simulink model "PID_MoreJoints1_6"  (R2018b)
settings: Solver=FixedStepDiscrete  StartTime=0.0  StopTime=Inf  FixedStep=0.001  RelTol=1e-3  EnableMultiTasking=on
undefined symbols (not defined in the file): DiscIntNeverNeededParam, J1, J2, J3, J4, J5, J6, J7, Motor_Current, Motor_Position, Motor_Velocity, q, qd, Send_GUIdata, Tau
libraries: c280xlib x14, simulink x11, dspsrcs4 x6, idelinklib_common x1
(part 1 of 4)
settings Model: ExtModeTrigDuration=8  Creator=Administrator  LastModifiedBy=Jeason
settings OptimizationCC: DefaultUnderspecifiedDataType=single  EnhancedBackFolding=on  PassReuseOutputArgsAs=Individual arguments  MaxStackSize=512  OptimizeBlockOrder=speed  DifferentSizesBufferReuse=on  OptimizationCustomize=off
settings DebuggingCC: InheritedTsInSrcMsg=none  MultiTaskDSMMsg=none  ParameterTunabilityLossMsg=error
settings HardwareCC: ProdBitPerChar=16  ProdBitPerInt=16  ProdBitPerPointer=32  ProdBitPerSizeT=32  ProdBitPerPtrDiffT=32  ProdLargestAtomicInteger=Integer  ProdLargestAtomicFloat=None  ProdWordSize=16  ProdLongLongMode=on  ProdHWDeviceType=Texas Instruments->C2000
settings SFSimCC: MATLABDynamicMemAlloc=off
settings RTWCC: SystemTargetFile=ert.tlc  HardwareBoard=TI Delfino F2833x  TemplateMakefile=ert_default_tmf  GenerateReport=on  Toolchain=Texas Instruments Code Composer Studio (C2000)  IncludeHyperlinkInReport=on  LaunchReport=on  GenerateTraceInfo=on  GenerateTraceReport=on  GenerateTraceReportSl=on  GenerateTraceReportSf=on  GenerateTraceReportEml=on
settings CodeAppCC: ForceParamTrailComments=on  IgnoreCustomStorageClasses=off  OperatorAnnotations=on  SimulinkDataObjDesc=on  SFDataObjDesc=on  InsertBlockDesc=on
settings ERTTargetCC: CodeReplacementLibrary=TI C28x

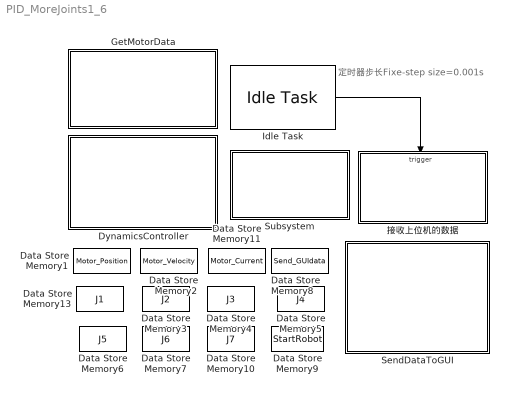
== system PID_MoreJoints1_6 ==
  note: 定时器步长Fixe-step size=0.001s
  Data Store Memory1 : DataStoreMemory  DataStoreName=Motor_Position  ReadBeforeWriteMsg=warning  WriteAfterWriteMsg=warning  WriteAfterReadMsg=warning  InitialValue=[0 0 0 0 0 0]  ShowAdditionalParam=off  OutDataTypeStr=int32
      settings: RTWStateStorageClass=ExportedGlobal
  Data Store Memory10 : DataStoreMemory  DataStoreName=J7  ReadBeforeWriteMsg=warning  WriteAfterWriteMsg=warning  WriteAfterReadMsg=warning  InitialValue=[0 0 0 0 0 0]  ShowAdditionalParam=off  OutDataTypeStr=double
      settings: RTWStateStorageClass=ExportedGlobal
  Data Store Memory11 : DataStoreMemory  DataStoreName=Motor_Current  ReadBeforeWriteMsg=warning  WriteAfterWriteMsg=warning  WriteAfterReadMsg=warning  InitialValue=[0 0 0 0 0 0]  ShowAdditionalParam=off  OutDataTypeStr=int32
      settings: RTWStateStorageClass=ExportedGlobal
  Data Store Memory13 : DataStoreMemory  DataStoreName=J1  ReadBeforeWriteMsg=warning  WriteAfterWriteMsg=warning  WriteAfterReadMsg=warning  InitialValue=[0 0 0 0 0 0]  ShowAdditionalParam=off  OutDataTypeStr=double
      settings: RTWStateStorageClass=ExportedGlobal
  Data Store Memory2 : DataStoreMemory  DataStoreName=Motor_Velocity  ReadBeforeWriteMsg=warning  WriteAfterWriteMsg=warning  WriteAfterReadMsg=warning  InitialValue=[0 0 0 0 0 0]  ShowAdditionalParam=off  OutDataTypeStr=int32
      settings: RTWStateStorageClass=ExportedGlobal
  Data Store Memory3 : DataStoreMemory  DataStoreName=J2  ReadBeforeWriteMsg=warning  WriteAfterWriteMsg=warning  WriteAfterReadMsg=warning  InitialValue=[0 0 0 0 0 0]  ShowAdditionalParam=off  OutDataTypeStr=double
      settings: RTWStateStorageClass=ExportedGlobal
  Data Store Memory4 : DataStoreMemory  DataStoreName=J3  ReadBeforeWriteMsg=warning  WriteAfterWriteMsg=warning  WriteAfterReadMsg=warning  InitialValue=[0 0 0 0 0 0]  ShowAdditionalParam=off  OutDataTypeStr=double
      settings: RTWStateStorageClass=ExportedGlobal
  Data Store Memory5 : DataStoreMemory  DataStoreName=J4  ReadBeforeWriteMsg=warning  WriteAfterWriteMsg=warning  WriteAfterReadMsg=warning  InitialValue=[0 0 0 0 0 0]  ShowAdditionalParam=off  OutDataTypeStr=double
      settings: RTWStateStorageClass=ExportedGlobal
  Data Store Memory6 : DataStoreMemory  DataStoreName=J5  ReadBeforeWriteMsg=warning  WriteAfterWriteMsg=warning  WriteAfterReadMsg=warning  InitialValue=[0 0 0 0 0 0]  ShowAdditionalParam=off  OutDataTypeStr=double
      settings: RTWStateStorageClass=ExportedGlobal
  Data Store Memory7 : DataStoreMemory  DataStoreName=J6  ReadBeforeWriteMsg=warning  WriteAfterWriteMsg=warning  WriteAfterReadMsg=warning  InitialValue=[0 0 0 0 0 0]  ShowAdditionalParam=off  OutDataTypeStr=double
      settings: RTWStateStorageClass=ExportedGlobal
  Data Store Memory8 : DataStoreMemory  DataStoreName=Send_GUIdata  ReadBeforeWriteMsg=warning  WriteAfterWriteMsg=warning  WriteAfterReadMsg=warning  InitialValue=zeros(1,18)  ShowAdditionalParam=off  OutDataTypeStr=double
      settings: RTWStateStorageClass=ExportedGlobal
  Data Store Memory9 : DataStoreMemory  DataStoreName=StartRobot  ReadBeforeWriteMsg=warning  WriteAfterWriteMsg=warning  WriteAfterReadMsg=warning  ShowAdditionalParam=off  OutDataTypeStr=uint16
      settings: RTWStateStorageClass=ExportedGlobal
  DynamicsController : Subsystem  Tag=Calculated_Data  Priority=2  TreatAsAtomicUnit=on  RTWFcnName=DynamicsController
      settings: RTWSystemCode=Nonreusable function  RTWFcnNameOpts=User specified  RTWFileNameOpts=Use function name
      mask Display:
      | color('red')
      | disp('六轴多关节\nPID算法动力学控制')
  GetMotorData : Subsystem  Tag=Get_Data  Priority=0  TreatAsAtomicUnit=on
      settings: RTWSystemCode=Nonreusable function
  Idle Task : idelinklib_common/Idle Task  tasknumbers=[0]  taskpriorities=100016  taskpreempts=[1]  showinput=off  simPriority=0
  SendDataToGUI : Subsystem  Priority=2  TreatAsAtomicUnit=on
      settings: RTWSystemCode=Nonreusable function
  Subsystem : Subsystem
      mask Display: disp('System\nInitialization');
  接收上位机的数据 : Subsystem  TreatAsAtomicUnit=on
  wires:
  Idle Task/1 -> 接收上位机的数据/Trigger

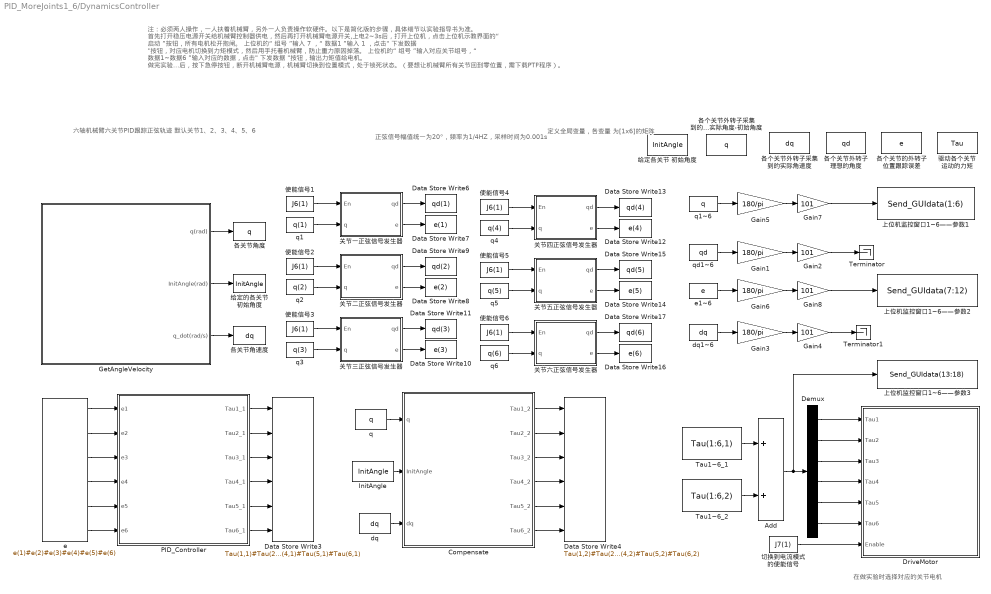
== system PID_MoreJoints1_6/DynamicsController ==
  note: 定义全局变量，各变量
      | 为[1x6]的矩阵
  note: 六轴机械臂六关节PID跟踪正弦轨迹
      | 默认关节1、2、3、4、5、6
  note: 在做实验时选择对应的关节电机
  note: 正弦信号幅值统一为20°，频率为1/4HZ，采样时间为0.001s
  note: 注：必须两人操作，一人扶着机械臂，另外一人负责操作软硬件。以下是简化版的步骤，具体细节以实验指导书为准。
      | 首先打开稳压电源开关给机械臂控制器供电，然后再打开机械臂电源开关,上电2~3s后，打开上位机，点击上位机示教界面的“ 启动 ”按钮，所有电机松开抱闸。
      | 上位机的“ 组号 ”输入 7 ，“ 数据1 ”输入 1 ，点击" 下发数据 "按钮，对应电机切换到力矩模式，然后用手托着机械臂，防止重力原因掉落。
      | 上位机的“ 组号 ”输入对应关节组号，“ 数据1~数据6 ”输入对应的数据，点击" 下发数据 "按钮，输出力矩值给电机。
      | 做完实验后，按下急停按钮，断开机械臂电源，机械臂切换到位置模式，处于锁死状态。（要想让机械臂所有关节回到零位置，需下载PTP程序）。
  Add : Sum
  Compensate : Subsystem  Priority=8  TreatAsAtomicUnit=on  RTWFcnName=Compensate
      settings: RTWSystemCode=Nonreusable function  RTWFcnNameOpts=User specified  RTWFileNameOpts=Use function name
  Data Store Write10 : DataStoreWrite  DataStoreName=e  DataStoreElements=e(3)
  Data Store Write11 : DataStoreWrite  DataStoreName=qd  DataStoreElements=qd(3)
  Data Store Write12 : DataStoreWrite  DataStoreName=e  DataStoreElements=e(4)
  Data Store Write13 : DataStoreWrite  DataStoreName=qd  DataStoreElements=qd(4)
  Data Store Write14 : DataStoreWrite  DataStoreName=e  DataStoreElements=e(5)
  Data Store Write15 : DataStoreWrite  DataStoreName=qd  DataStoreElements=qd(5)
  Data Store Write16 : DataStoreWrite  DataStoreName=e  DataStoreElements=e(6)
  Data Store Write17 : DataStoreWrite  DataStoreName=qd  DataStoreElements=qd(6)
  Data Store Write3 : DataStoreWrite  DataStoreName=Tau  DataStoreElements=Tau(1,1)#Tau(2,1)#Tau(3,1)#Tau(4,1)#Tau(5,1)#Tau(6,1)
  Data Store Write4 : DataStoreWrite  DataStoreName=Tau  DataStoreElements=Tau(1,2)#Tau(2,2)#Tau(3,2)#Tau(4,2)#Tau(5,2)#Tau(6,2)
  Data Store Write6 : DataStoreWrite  DataStoreName=qd  DataStoreElements=qd(1)
  Data Store Write7 : DataStoreWrite  DataStoreName=e  DataStoreElements=e(1)
  Data Store Write8 : DataStoreWrite  DataStoreName=e  DataStoreElements=e(2)
  Data Store Write9 : DataStoreWrite  DataStoreName=qd  DataStoreElements=qd(2)
  Demux : Demux  Outputs=6
  DriveMotor : Subsystem  TreatAsAtomicUnit=on  RTWFcnName=DrivrMotor  mask(DriverMotor){Motor1=on, Motor2=on, Motor3=on, Motor4=on, Motor5=on, Motor6=on}
      mask help:
      | 当其中一个Motor勾选时，表示将力矩输出给对应的电机；如果不勾选时，表示对应的电机不工作。
      | 比如：如果做单关节实验时，哪个电机要做实验就勾选对应的电机，其他电机一定要不勾选。
      | 关节1~3为CANB,关节4~6为CANA,驱动邮箱号为7~12。输入量的范围限定在-900~900。
      settings: RTWSystemCode=Nonreusable function  RTWFcnNameOpts=User specified  RTWFileNameOpts=Use function name
      mask Callback Motor1:
      | vssBlk1 = [gcb, '/BottomDriver/Joint1'];
      | choice1 = get_param(gcb,'Motor1');
      | if strcmp(choice1,'off')
      |         set_param(vssBlk1, 'Commented','on');
      |     else
      |         set_param(vssBlk1, 'Commented','off');
      | end
      | clear choice1 vssBlk1;
      mask Callback Motor2:
      | vssBlk2 = [gcb, '/BottomDriver/Joint2'];
      | choice2 = get_param(gcb,'Motor2');
      | if strcmp(choice2,'off')
      |         set_param(vssBlk2, 'Commented','on');
      |     else
      |         set_param(vssBlk2, 'Commented','off');
      | end
      | clear choice2 vssBlk2;
      mask Callback Motor3:
      | vssBlk3 = [gcb, '/BottomDriver/Joint3'];
      | choice3 = get_param(gcb,'Motor3');
      | if strcmp(choice3,'off')
      |         set_param(vssBlk3, 'Commented','on');
      |     else
      |         set_param(vssBlk3, 'Commented','off');
      | end
      | clear choice3 vssBlk3;
      mask Callback Motor4:
      | vssBlk4 = [gcb, '/BottomDriver/Joint4'];
      | choice4 = get_param(gcb,'Motor4');
      | if strcmp(choice4,'off')
      |         set_param(vssBlk4, 'Commented','on');
      |     else
      |         set_param(vssBlk4, 'Commented','off');
      | end
      | clear choice4 vssBlk4;
      mask Callback Motor5:
      | vssBlk5 = [gcb, '/BottomDriver/Joint5'];
      | choice5 = get_param(gcb,'Motor5');
      | if strcmp(choice5,'off')
      |         set_param(vssBlk5, 'Commented','on');
      |     else
      |         set_param(vssBlk5, 'Commented','off');
      | end
      | clear choice5 vssBlk5;
      mask Callback Motor6:
      | vssBlk6 = [gcb, '/BottomDriver/Joint6'];
      | choice6 = get_param(gcb,'Motor6');
      | if strcmp(choice6,'off')
      |         set_param(vssBlk6, 'Commented','on');
      |     else
      |         set_param(vssBlk6, 'Commented','off');
      | end
      | clear choice6 vssBlk6;
      mask Display:
      | disp('DriverMotor');
      | port_label('input', 1, 'Tau1');
      | port_label('input', 2, 'Tau2');
      | port_label('input', 3, 'Tau3');
      | port_label('input', 4, 'Tau4');
      | port_label('input', 5, 'Tau5');
      | port_label('input', 6, 'Tau6');
      | port_label('input', 7, 'Enable');
  Gain{1,3,5..6} (4 alike) : Gain  Gain=180/pi
  Gain{2,4,7..8} (4 alike) : Gain  Gain=101
  GetAngleVelocity : Subsystem  Priority=0  TreatAsAtomicUnit=on  RTWFcnName=GetAngleVelocity
      settings: RTWSystemCode=Nonreusable function  RTWFcnNameOpts=User specified  RTWFileNameOpts=Use function name
  InitAngle : DataStoreRead  DataStoreName=InitAngle
  PID_Controller : Subsystem  Priority=7  TreatAsAtomicUnit=on  RTWFcnName=PID_Controller
      settings: RTWSystemCode=Nonreusable function  RTWFcnNameOpts=User specified  RTWFileNameOpts=Use function name
  Tau1~6_1 : DataStoreRead  DataStoreName=Tau  DataStoreElements=Tau(1:6,1)
  Tau1~6_2 : DataStoreRead  DataStoreName=Tau  DataStoreElements=Tau(1:6,2)
  Terminator : Terminator
  Terminator1 : Terminator
  dq : DataStoreRead  DataStoreName=dq
  dq1~6 : DataStoreRead  DataStoreName=dq
  e : DataStoreRead  DataStoreName=e  DataStoreElements=e(1)#e(2)#e(3)#e(4)#e(5)#e(6)
  e1~6 : DataStoreRead  DataStoreName=e
  q : DataStoreRead  DataStoreName=q
  q1 : DataStoreRead  DataStoreName=q  DataStoreElements=q(1)
  q1~6 : DataStoreRead  DataStoreName=q
  q2 : DataStoreRead  DataStoreName=q  DataStoreElements=q(2)
  q3 : DataStoreRead  DataStoreName=q  DataStoreElements=q(3)
  q4 : DataStoreRead  DataStoreName=q  DataStoreElements=q(4)
  q5 : DataStoreRead  DataStoreName=q  DataStoreElements=q(5)
  q6 : DataStoreRead  DataStoreName=q  DataStoreElements=q(6)
  qd1~6 : DataStoreRead  DataStoreName=qd
  上位机监控窗口1~6——参数1 : DataStoreWrite  DataStoreName=Send_GUIdata  DataStoreElements=Send_GUIdata(1:6)
  上位机监控窗口1~6——参数2 : DataStoreWrite  DataStoreName=Send_GUIdata  DataStoreElements=Send_GUIdata(7:12)
  上位机监控窗口1~6——参数3 : DataStoreWrite  DataStoreName=Send_GUIdata  DataStoreElements=Send_GUIdata(13:18)
  使能信号{1..6} (6 alike) : DataStoreRead  DataStoreName=J6  DataStoreElements=J6(1)
  关节一正弦信号发生器 : Subsystem  Priority=1  TreatAsAtomicUnit=on  RTWFcnName=SineSignal
      settings: RTWFcnNameOpts=User specified  RTWFileNameOpts=Use function name
  关节三正弦信号发生器 : Subsystem  Priority=3  TreatAsAtomicUnit=on  RTWFcnName=SineSignal
      settings: RTWFcnNameOpts=User specified  RTWFileNameOpts=Use function name
  关节二正弦信号发生器 : Subsystem  Priority=2  TreatAsAtomicUnit=on  RTWFcnName=SineSignal
      settings: RTWFcnNameOpts=User specified  RTWFileNameOpts=Use function name
  关节五正弦信号发生器 : Subsystem  Priority=5  TreatAsAtomicUnit=on  RTWFcnName=SineSignal
      settings: RTWFcnNameOpts=User specified  RTWFileNameOpts=Use function name
  关节六正弦信号发生器 : Subsystem  Priority=6  TreatAsAtomicUnit=on  RTWFcnName=SineSignal
      settings: RTWFcnNameOpts=User specified  RTWFileNameOpts=Use function name
  关节四正弦信号发生器 : Subsystem  Priority=4  TreatAsAtomicUnit=on  RTWFcnName=SineSignal
      settings: RTWFcnNameOpts=User specified  RTWFileNameOpts=Use function name
  切换到电流模式 的使能信号 : DataStoreRead  DataStoreName=J7  DataStoreElements=J7(1)
  各个关节外转子 理想的角度 : DataStoreMemory  DataStoreName=qd  ReadBeforeWriteMsg=warning  WriteAfterWriteMsg=warning  WriteAfterReadMsg=warning  InitialValue=zeros(1,6)  ShowAdditionalParam=off  OutDataTypeStr=double
      settings: RTWStateStorageClass=ExportedGlobal
  各个关节外转子采集 到的实际角度-初始角度 : DataStoreMemory  DataStoreName=q  ReadBeforeWriteMsg=warning  WriteAfterWriteMsg=warning  WriteAfterReadMsg=warning  InitialValue=zeros(1,6)  ShowAdditionalParam=off  OutDataTypeStr=double
      settings: RTWStateStorageClass=ExportedGlobal
  各个关节外转子采集 到的实际角速度 : DataStoreMemory  DataStoreName=dq  ReadBeforeWriteMsg=warning  WriteAfterWriteMsg=warning  WriteAfterReadMsg=warning  InitialValue=zeros(1,6)  ShowAdditionalParam=off  OutDataTypeStr=double
      settings: RTWStateStorageClass=ExportedGlobal
  各个关节的外转子 位置跟踪误差 : DataStoreMemory  DataStoreName=e  ReadBeforeWriteMsg=warning  WriteAfterWriteMsg=warning  WriteAfterReadMsg=warning  InitialValue=zeros(1,6)  ShowAdditionalParam=off  OutDataTypeStr=double
      settings: RTWStateStorageClass=ExportedGlobal
  各关节角度 : DataStoreWrite  DataStoreName=q
  各关节角速度 : DataStoreWrite  DataStoreName=dq
  给定各关节 初始角度 : DataStoreMemory  DataStoreName=InitAngle  ReadBeforeWriteMsg=warning  WriteAfterWriteMsg=warning  WriteAfterReadMsg=warning  InitialValue=zeros(1,6)  ShowAdditionalParam=off  OutDataTypeStr=double
      settings: RTWStateStorageClass=ExportedGlobal
  给定的各关节 初始角度 : DataStoreWrite  DataStoreName=InitAngle
  驱动各个关节 运动的力矩 : DataStoreMemory  DataStoreName=Tau  ReadBeforeWriteMsg=warning  WriteAfterWriteMsg=warning  WriteAfterReadMsg=warning  InitialValue=zeros(6,2)  ShowAdditionalParam=off  OutDataTypeStr=double
      settings: RTWStateStorageClass=ExportedGlobal
  wires:
  使能信号1/1 -> 关节一正弦信号发生器/1(En)
  使能信号2/1 -> 关节二正弦信号发生器/1(En)
  使能信号3/1 -> 关节三正弦信号发生器/1(En)
  使能信号4/1 -> 关节四正弦信号发生器/1(En)
  使能信号5/1 -> 关节五正弦信号发生器/1(En)
  使能信号6/1 -> 关节六正弦信号发生器/1(En)
  关节一正弦信号发生器/1(qd) -> Data Store Write6/1
  关节二正弦信号发生器/1(qd) -> Data Store Write9/1
  关节三正弦信号发生器/1(qd) -> Data Store Write11/1
  关节四正弦信号发生器/1(qd) -> Data Store Write13/1
  关节五正弦信号发生器/1(qd) -> Data Store Write15/1
  关节六正弦信号发生器/1(qd) -> Data Store Write17/1
  关节一正弦信号发生器/2(e) -> Data Store Write7/1
  关节二正弦信号发生器/2(e) -> Data Store Write8/1
  关节三正弦信号发生器/2(e) -> Data Store Write10/1
  关节四正弦信号发生器/2(e) -> Data Store Write12/1
  关节五正弦信号发生器/2(e) -> Data Store Write14/1
  关节六正弦信号发生器/2(e) -> Data Store Write16/1
  q1/1 -> 关节一正弦信号发生器/2(q)
  q2/1 -> 关节二正弦信号发生器/2(q)
  q3/1 -> 关节三正弦信号发生器/2(q)
  q4/1 -> 关节四正弦信号发生器/2(q)
  q5/1 -> 关节五正弦信号发生器/2(q)
  q6/1 -> 关节六正弦信号发生器/2(q)
  e/1 -> PID_Controller/1(e1)
  e/2 -> PID_Controller/2(e2)
  e/3 -> PID_Controller/3(e3)
  e/4 -> PID_Controller/4(e4)
  e/5 -> PID_Controller/5(e5)
  e/6 -> PID_Controller/6(e6)
  PID_Controller/1(Tau1_1) -> Data Store Write3/1
  PID_Controller/2(Tau2_1) -> Data Store Write3/2
  PID_Controller/3(Tau3_1) -> Data Store Write3/3
  PID_Controller/4(Tau4_1) -> Data Store Write3/4
  PID_Controller/5(Tau5_1) -> Data Store Write3/5
  PID_Controller/6(Tau6_1) -> Data Store Write3/6
  Tau1~6_1/1 -> Add/1
  Tau1~6_2/1 -> Add/2
  Add/1 -> 上位机监控窗口1~6——参数3/1, Demux/1
  Demux/6 -> DriveMotor/6(Tau6)
  Demux/5 -> DriveMotor/5(Tau5)
  Demux/4 -> DriveMotor/4(Tau4)
  Demux/3 -> DriveMotor/3(Tau3)
  Demux/2 -> DriveMotor/2(Tau2)
  Demux/1 -> DriveMotor/1(Tau1)
  切换到电流模式 的使能信号/1 -> DriveMotor/7(Enable)
  q1~6/1 -> Gain5/1
  Gain5/1 -> Gain7/1
  Gain1/1 -> Gain2/1
  qd1~6/1 -> Gain1/1
  Gain3/1 -> Gain4/1
  dq1~6/1 -> Gain3/1
  Gain6/1 -> Gain8/1
  e1~6/1 -> Gain6/1
  Gain7/1 -> 上位机监控窗口1~6——参数1/1
  Gain8/1 -> 上位机监控窗口1~6——参数2/1
  Gain4/1 -> Terminator1/1
  q/1 -> Compensate/1(q)
  dq/1 -> Compensate/3(dq)
  Gain2/1 -> Terminator/1
  Compensate/1(Tau1_2) -> Data Store Write4/1
  Compensate/2(Tau2_2) -> Data Store Write4/2
  Compensate/3(Tau3_2) -> Data Store Write4/3
  Compensate/4(Tau4_2) -> Data Store Write4/4
  Compensate/5(Tau5_2) -> Data Store Write4/5
  Compensate/6(Tau6_2) -> Data Store Write4/6
  GetAngleVelocity/2(InitAngle(rad)) -> 给定的各关节 初始角度/1
  GetAngleVelocity/3(q_dot(rad/s)) -> 各关节角速度/1
  GetAngleVelocity/1(q(rad)) -> 各关节角度/1
  InitAngle/1 -> Compensate/2(InitAngle)

== system PID_MoreJoints1_6/GetMotorData ==
  note: 获取关节电流、 角速度、 角度信息
  CANA_284_24 : Subsystem  Priority=4  TreatAsAtomicUnit=on
      settings: RTWSystemCode=Nonreusable function
      mask Display:
      | color('WHITE')
      | disp('JOINT4\n数据读取')
  CANA_285_25 : Subsystem  Priority=5  TreatAsAtomicUnit=on
      settings: RTWSystemCode=Nonreusable function
      mask Display:
      | color('WHITE')
      | disp('JOINT5\n数据读取')
  CANA_286_26 : Subsystem  Priority=6  TreatAsAtomicUnit=on
      settings: RTWSystemCode=Nonreusable function
      mask Display:
      | color('WHITE')
      | disp('JOINT6\n数据读取')
  CANB_281_21 : Subsystem  Priority=1  TreatAsAtomicUnit=on
      settings: RTWSystemCode=Nonreusable function
      mask Display:
      | color('WHITE')
      | disp('JOINT1\n数据读取')
  CANB_282_22 : Subsystem  Priority=2  TreatAsAtomicUnit=on
      settings: RTWSystemCode=Nonreusable function
      mask Display:
      | color('white')
      | disp('JOINT2\n数据读取')
  CANB_283_23 : Subsystem  Priority=3  TreatAsAtomicUnit=on
      settings: RTWSystemCode=Nonreusable function
      mask Display:
      | color('white')
      | disp('JOINT3\n数据读取')

== system PID_MoreJoints1_6/SendDataToGUI ==
  note: Upper limit=9
  note: 发送数据给上位机
  note: 定时器步长Fixe-step size=0.001s,
      | 每10ms发送一次数据给上位机
  " " : Subsystem
  Constant : Constant  Value=true  OutDataTypeStr=boolean
  Constant1 : Constant  Value=false  OutDataTypeStr=boolean
  Switch : Switch  Criteria=u2 > Threshold
  广播周期 : simulink/Sources/Counter Limited  uplimit=9  tsamp=-1
  wires:
  Switch/1 -> " "/Enable
  广播周期/1 -> Switch/2
  Constant1/1 -> Switch/1
  Constant/1 -> Switch/3

== system PID_MoreJoints1_6/Subsystem ==
  Model Header : Subsystem  mask(Model Header){ShowInLibBrowser=0}
      mask prompts: ShowInLibBrowser "Simulink:masks:CustCodeMaskParam1_MP"
      settings: CopyFcn=cccopyfcn(gcb)  OpenFcn=ccopenfcn('Model Header')
      mask Help: eval('feval(''rtwprivate'',''rtwhelpview'',''rtw_model_header_block'')');
      mask Display: disp('Model\nHeader');
  Model Source : Subsystem  mask(Model Source){ShowInLibBrowser=0}
      mask prompts: ShowInLibBrowser "Simulink:masks:CustCodeMaskParam1_MP"
      settings: CopyFcn=cccopyfcn(gcb)  OpenFcn=ccopenfcn('Model Source')
      mask Help: eval('feval(''rtwprivate'',''rtwhelpview'',''rtw_model_source_block'')');
      mask Display: disp('Model\nSource');
  System Initialize : Subsystem  mask(System Initialize){ShowInLibBrowser=0}
      mask prompts: ShowInLibBrowser "Simulink:masks:CustCodeMaskParam1_MP"
      settings: CopyFcn=cccopyfcn(gcb)  OpenFcn=ccopenfcn('System Initialize Function')
      mask Help: eval('feval(''rtwprivate'',''rtwhelpview'',''rtw_sys_initialize_block'')');
      mask Display: disp('System\nInitialize');

== system PID_MoreJoints1_6/接收上位机的数据 ==
  note: 接收上位机数据
  function : TriggerPort  TriggerType=function-call  VariantControl=Variant
  0x0080 : simulink/Logic and Bit Operations/Compare To Constant  relop===  const=hex2dec('0080')  OutDataTypeStr=boolean
  0x88 : simulink/Logic and Bit Operations/Compare To Constant  relop===  const=hex2dec('0088')  OutDataTypeStr=boolean
  Compare To Constant1 : simulink/Logic and Bit Operations/Compare To Constant  relop===  const=hex2dec('0001')  OutDataTypeStr=boolean
  Compare To Constant2 : simulink/Logic and Bit Operations/Compare To Constant  relop===  const=hex2dec('0001')  OutDataTypeStr=boolean
  Data Store Read : DataStoreRead  DataStoreName=PTX
  Data Store Write2 : DataStoreWrite  DataStoreName=StartRobot
  Data Type Conversion : DataTypeConversion  OutDataTypeStr=int16
  Data Type Conversion3 : DataTypeConversion  OutDataTypeStr=double
  Data Type Conversion4 : DataTypeConversion  OutDataTypeStr=uint16
  Demux1 : Demux  Outputs=9
  Logical Operator : Logic  Inputs=4  AllPortsSameDT=off  OutDataTypeStr=boolean
  Mux1 : Mux  Inputs=6
  Subsystem : Subsystem
  Terminator3 : Terminator
  消息使能 : DataStoreMemory  DataStoreName=PTX  ReadBeforeWriteMsg=warning  WriteAfterWriteMsg=warning  WriteAfterReadMsg=warning  InitialValue=true  ShowAdditionalParam=off  OutDataTypeStr=boolean
  获取用户命令 : Subsystem  Priority=1  TreatAsAtomicUnit=on
      settings: RTWSystemCode=Nonreusable function
  wires:
  Compare To Constant2/1 -> Logical Operator/4
  Compare To Constant1/1 -> Logical Operator/3
  Data Store Read/1 -> Logical Operator/2
  Logical Operator/1 -> Data Type Conversion4/1
  0x0080/1 -> Logical Operator/1
  Demux1/4 -> Mux1/2, Compare To Constant2/1
  Demux1/3 -> Mux1/1, Compare To Constant1/1
  Demux1/1 -> 0x0080/1, 0x88/1
  获取用户命令/1(消息) -> Demux1/1
  Demux1/5 -> Mux1/3
  Demux1/6 -> Mux1/4
  Demux1/9 -> Terminator3/1
  Demux1/7 -> Mux1/5
  Demux1/8 -> Mux1/6
  Mux1/1 -> Data Type Conversion/1
  Data Type Conversion/1 -> Data Type Conversion3/1
  Data Type Conversion4/1 -> Data Store Write2/1
  Demux1/2 -> Subsystem/1(组号)
  Data Type Conversion3/1 -> Subsystem/2(数据)
  0x88/1 -> Subsystem/Enable

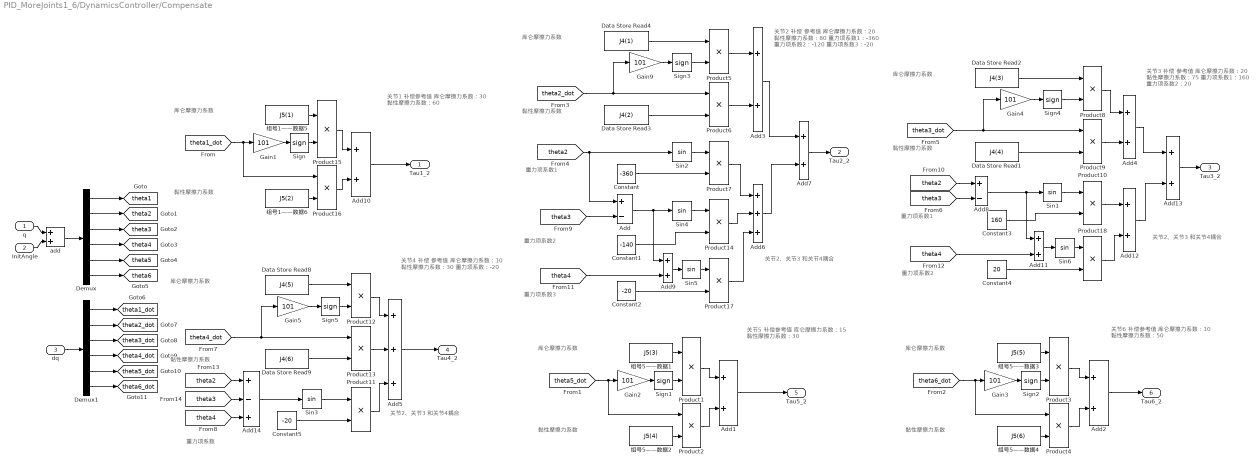
== system PID_MoreJoints1_6/DynamicsController/Compensate ==
  note: 关节1 补偿参考值
      | 库仑摩擦力系数：30
      | 黏性摩擦力系数：60
  note: 关节6 补偿参考值
      | 库仑摩擦力系数：10
      | 黏性摩擦力系数：50
  note: 库仑摩擦力系数
  note: 关节5 补偿参考值
      | 库仑摩擦力系数：15
      | 黏性摩擦力系数：30
  note: 黏性摩擦力系数
  note: 库仑摩擦力系数
  note: 黏性摩擦力系数
  note: 库仑摩擦力系数
  note: 黏性摩擦力系数
  note: 黏性摩擦力系数
  note: 关节2 补偿 参考值
      | 库仑摩擦力系数：20
      | 黏性摩擦力系数：80
      | 重力项系数1：-360
      | 重力项系数2：-120
      | 重力项系数3：-20
  note: 重力项系数1
  note: 库仑摩擦力系数
  note: 黏性摩擦力系数
  note: 关节3 补偿 参考值
      | 库仑摩擦力系数：20
      | 黏性摩擦力系数：75
      | 重力项系数1：160
      | 重力项系数2：20
  note: 重力项系数1
  note: 库仑摩擦力系数
  note: 黏性摩擦力系数
  note: 关节4 补偿 参考值
      | 库仑摩擦力系数：10
      | 黏性摩擦力系数：30
      | 重力项系数：-20
  note: 重力项系数
  note: 库仑摩擦力系数
  note: 关节2、关节3
      | 和关节4耦合
  note: 重力项系数2
  note: 重力项系数3
  note: 关节2、关节3
      | 和关节4耦合
  note: 关节2、关节3
      | 和关节4耦合
  note: 重力项系数2
  q : Inport
  InitAngle : Inport  Port=2
  dq : Inport  Port=3
  Add : Sum  Inputs=+-
  Add{1..2,9..11} (5 alike) : Sum
  Add{3..4,7,12..13} (5 alike) : Sum  Inputs=2
  Add14 : Sum  Inputs=+-+
  Add5 : Sum  Inputs=+++
  Add6 : Sum  Inputs=3
  Add8 : Sum  Inputs=+-
  Constant : Constant  Value=-360
  Constant1 : Constant  Value=-140
  Constant2 : Constant  Value=-20
  Constant3 : Constant  Value=160
  Constant4 : Constant  Value=20
  Constant5 : Constant  Value=-20
  Data Store Read1 : DataStoreRead  DataStoreName=J4  DataStoreElements=J4(4)
  Data Store Read2 : DataStoreRead  DataStoreName=J4  DataStoreElements=J4(3)
  Data Store Read3 : DataStoreRead  DataStoreName=J4  DataStoreElements=J4(2)
  Data Store Read4 : DataStoreRead  DataStoreName=J4  DataStoreElements=J4(1)
  Data Store Read8 : DataStoreRead  DataStoreName=J4  DataStoreElements=J4(5)
  Data Store Read9 : DataStoreRead  DataStoreName=J4  DataStoreElements=J4(6)
  Demux : Demux  Outputs=6
  Demux1 : Demux  Outputs=6
  Gain{1..5,9} (6 alike) : Gain  Gain=101
  Product{1,3,5,7..8,10..12,14..15,17..18} (12 alike) : Product
  Product{2,4,6,9,13,16} (6 alike) : Product  OutDataTypeStr=double
  Sign{,1..5} (6 alike) : Signum
  Sin{1..6} (6 alike) : Trigonometry
  add : Sum
  组号1——数据5 : DataStoreRead  DataStoreName=J5  DataStoreElements=J5(1)
  组号1——数据6 : DataStoreRead  DataStoreName=J5  DataStoreElements=J5(2)
  组号5——数据1 : DataStoreRead  DataStoreName=J5  DataStoreElements=J5(3)
  组号5——数据2 : DataStoreRead  DataStoreName=J5  DataStoreElements=J5(4)
  组号5——数据3 : DataStoreRead  DataStoreName=J5  DataStoreElements=J5(5)
  组号5——数据4 : DataStoreRead  DataStoreName=J5  DataStoreElements=J5(6)
  Tau1_2 : Outport
  Tau2_2 : Outport  Port=2
  Tau3_2 : Outport  Port=3
  Tau4_2 : Outport  Port=4
  Tau5_2 : Outport  Port=5
  Tau6_2 : Outport  Port=6
  tag scope: theta1=global, theta1_dot=global, theta2=global, theta2_dot=global, theta3=global, theta3_dot=global, theta4=global, theta4_dot=global, theta5=global, theta5_dot=global, theta6=global, theta6_dot=global
  wires:
  [theta1_dot] -> Product16/1, Gain1/1
  Sign/1 -> Product15/2
  Product16/1 -> Add10/2
  Product15/1 -> Add10/1
  Gain1/1 -> Sign/1
  组号1——数据5/1 -> Product15/1
  Add10/1 -> Tau1_2/1
  组号1——数据6/1 -> Product16/2
  组号5——数据2/1 -> Product2/2
  Add1/1 -> Tau5_2/1
  组号5——数据1/1 -> Product1/1
  Gain2/1 -> Sign1/1
  Product1/1 -> Add1/1
  Product2/1 -> Add1/2
  Sign1/1 -> Product1/2
  [theta5_dot] -> Gain2/1, Product2/1
  [theta6_dot] -> Product4/1, Gain3/1
  Sign2/1 -> Product3/2
  Product4/1 -> Add2/2
  Product3/1 -> Add2/1
  Gain3/1 -> Sign2/1
  组号5——数据3/1 -> Product3/1
  Add2/1 -> Tau6_2/1
  组号5——数据4/1 -> Product4/2
  Gain9/1 -> Sign3/1
  Data Store Read4/1 -> Product5/1
  Product7/1 -> Add6/1
  Sin2/1 -> Product7/1
  Product5/1 -> Add3/1
  Product6/1 -> Add3/2
  [theta2] -> Add/1, Sin2/1
  Data Store Read3/1 -> Product6/2
  Constant/1 -> Product7/2
  [theta2_dot] -> Gain9/1, Product6/1
  Sign3/1 -> Product5/2
  Add3/1 -> Add7/1
  add/1 -> Demux/1
  dq/1 -> Demux1/1
  Demux/1 -> [theta1]
  Demux/2 -> [theta2]
  Demux/3 -> [theta3]
  Demux/4 -> [theta4]
  Demux/5 -> [theta5]
  Demux/6 -> [theta6]
  Demux1/1 -> [theta1_dot]
  Demux1/2 -> [theta2_dot]
  Demux1/3 -> [theta3_dot]
  Demux1/4 -> [theta4_dot]
  Demux1/5 -> [theta5_dot]
  Demux1/6 -> [theta6_dot]
  Sign4/1 -> Product8/2
  [theta3_dot] -> Product9/1, Gain4/1
  Constant3/1 -> Product10/2
  Data Store Read1/1 -> Product9/2
  Product9/1 -> Add4/2
  Product8/1 -> Add4/1
  Sin1/1 -> Product10/1
  Product10/1 -> Add12/1
  Data Store Read2/1 -> Product8/1
  Gain4/1 -> Sign4/1
  Gain5/1 -> Sign5/1
  Data Store Read8/1 -> Product12/1
  Product11/1 -> Add5/3
  Sin3/1 -> Product11/1
  Product12/1 -> Add5/1
  Product13/1 -> Add5/2
  [theta2] -> Add14/1
  Data Store Read9/1 -> Product13/2
  [theta4_dot] -> Gain5/1, Product13/1
  Sign5/1 -> Product12/2
  Add5/1 -> Tau4_2/1
  [theta3] -> Add/2
  Add/1 -> Add9/1, Sin4/1
  Sin4/1 -> Product14/1
  Constant1/1 -> Product14/2
  Product14/1 -> Add6/2
  Add6/1 -> Add7/2
  Add7/1 -> Tau2_2/1
  [theta2] -> Add8/1
  [theta3] -> Add8/2
  [theta4] -> Add9/2
  Add9/1 -> Sin5/1
  Sin5/1 -> Product17/1
  Constant2/1 -> Product17/2
  Product17/1 -> Add6/3
  Product18/1 -> Add12/2
  Constant4/1 -> Product18/2
  Sin6/1 -> Product18/1
  Add11/1 -> Sin6/1
  [theta4] -> Add11/2
  Add8/1 -> Add11/1, Sin1/1
  Add4/1 -> Add13/1
  Add12/1 -> Add13/2
  Add13/1 -> Tau3_2/1
  [theta3] -> Add14/2
  [theta4] -> Add14/3
  Add14/1 -> Sin3/1
  Constant5/1 -> Product11/2
  InitAngle/1 -> add/2
  q/1 -> add/1

== system PID_MoreJoints1_6/DynamicsController/DriveMotor ==
  Tau1 : Inport
  Tau2 : Inport  Port=2
  Tau3 : Inport  Port=3
  Tau4 : Inport  Port=4
  Tau5 : Inport  Port=5
  Tau6 : Inport  Port=6
  Enable : Inport  Port=7
  BottomDriver : Subsystem
  Data Store Memory1 : DataStoreMemory  DataStoreName=TXD  ReadBeforeWriteMsg=warning  WriteAfterWriteMsg=warning  WriteAfterReadMsg=warning  InitialValue=[0]  ShowAdditionalParam=off  OutDataTypeStr=uint8
      settings: RTWStateStorageClass=ExportedGlobal
  Data Store Read4 : DataStoreRead  DataStoreName=TXD
  Saturation{1..6} (6 alike) : Saturate  UpperLimit=900  LowerLimit=-900
  驱动器指令 : Subsystem  TreatAsAtomicUnit=on
      settings: RTWSystemCode=Nonreusable function
  wires:
  Data Store Read4/1 -> BottomDriver/Enable
  驱动器指令/4(MSG4) -> BottomDriver/4(JOINT4)
  驱动器指令/3(MSG3) -> BottomDriver/3(JOINT3)
  驱动器指令/1(MSG1) -> BottomDriver/1(JOINT1)
  驱动器指令/2(MSG2) -> BottomDriver/2(JOINT2)
  Enable/1 -> 驱动器指令/7(Enable)
  驱动器指令/5(MSG5) -> BottomDriver/5(JOINT5)
  Saturation2/1 -> 驱动器指令/1(Current1)
  Saturation1/1 -> 驱动器指令/2(Current2)
  Saturation3/1 -> 驱动器指令/3(Current3)
  Saturation4/1 -> 驱动器指令/4(Current4)
  Saturation5/1 -> 驱动器指令/5(Current5)
  Tau1/1 -> Saturation2/1
  Tau2/1 -> Saturation1/1
  Tau3/1 -> Saturation3/1
  Tau4/1 -> Saturation4/1
  Tau5/1 -> Saturation5/1
  驱动器指令/6(MSG6) -> BottomDriver/6(JOINT6)
  Tau6/1 -> Saturation6/1
  Saturation6/1 -> 驱动器指令/6(Current6)

== system PID_MoreJoints1_6/DynamicsController/GetAngleVelocity ==
  GetAngle1 : Subsystem  TreatAsAtomicUnit=on  mask(获取电机外转子角度(rad)){JJoint=1, InitAngle=0}
      mask prompts: JJoint "选择关节电机"; InitAngle "给定初始角度(deg)"
      mask help:
      | 给定初始角度：假设在数学建模时，设定连杆在水平位置为0°，而机械臂每个关节在出厂时都设定在竖直位置为0°，那么这里就需要给定一个偏置值90°/-90°，默认设为0。
      | 注：关节3因为结构原因实际获取到的角度的正负和标签贴的方向相反。
      | Angle(rad)=电机外转子的实际角度值-给定的初始角度值
      | InitAngle(rad)=给定的初始角度值
      mask TypeOptions JJoint: 1 | 2 | 3 | 4 | 5 | 6
      mask Display:
      | choice1 = get_param(gcb,'JJoint');
      | color('black');
      | switch choice1
      |     case '1'
      |         disp('获取关节1电机\n外转子角度(rad)');
      |     case '2'
      |         disp('获取关节2电机\n外转子角度(rad)');
      |     case '3'
      |         disp('获取关节3电机\n外转子角度(rad)');
      |     case '4'
      |         disp('获取关节4电机\n外转子角度(rad)');
      |     case '5'
      |         disp('获取关节5电机\n外转子角度(rad)');
      |     case '6'
      |         disp('获取关节6电机\n外转子角度(rad)');
      | end
      | color('black');
      | port_label('output', 1, 'Angle');
      | port_label('output', 2, 'InitAngle');
      | clear choice1;
  GetAngle2 : Subsystem  TreatAsAtomicUnit=on  mask(获取电机外转子角度(rad)){JJoint=2, InitAngle=0}
      mask prompts: JJoint "选择关节电机"; InitAngle "给定初始角度(deg)"
      mask help:
      | 给定初始角度：假设在数学建模时，设定连杆在水平位置为0°，而机械臂每个关节在出厂时都设定在竖直位置为0°，那么这里就需要给定一个偏置值90°/-90°，默认设为0。
      | 注：关节3因为结构原因实际获取到的角度的正负和标签贴的方向相反。
      | Angle(rad)=电机外转子的实际角度值-给定的初始角度值
      | InitAngle(rad)=给定的初始角度值
      mask TypeOptions JJoint: 1 | 2 | 3 | 4 | 5 | 6
      mask Display:
      | choice1 = get_param(gcb,'JJoint');
      | color('black');
      | switch choice1
      |     case '1'
      |         disp('获取关节1电机\n外转子角度(rad)');
      |     case '2'
      |         disp('获取关节2电机\n外转子角度(rad)');
      |     case '3'
      |         disp('获取关节3电机\n外转子角度(rad)');
      |     case '4'
      |         disp('获取关节4电机\n外转子角度(rad)');
      |     case '5'
      |         disp('获取关节5电机\n外转子角度(rad)');
      |     case '6'
      |         disp('获取关节6电机\n外转子角度(rad)');
      | end
      | color('black');
      | port_label('output', 1, 'Angle');
      | port_label('output', 2, 'InitAngle');
      | clear choice1;
  GetAngle3 : Subsystem  TreatAsAtomicUnit=on  mask(获取电机外转子角度(rad)){JJoint=3, InitAngle=0}
      mask prompts: JJoint "选择关节电机"; InitAngle "给定初始角度(deg)"
      mask help:
      | 给定初始角度：假设在数学建模时，设定连杆在水平位置为0°，而机械臂每个关节在出厂时都设定在竖直位置为0°，那么这里就需要给定一个偏置值90°/-90°，默认设为0。
      | 注：关节3因为结构原因实际获取到的角度的正负和标签贴的方向相反。
      | Angle(rad)=电机外转子的实际角度值-给定的初始角度值
      | InitAngle(rad)=给定的初始角度值
      mask TypeOptions JJoint: 1 | 2 | 3 | 4 | 5 | 6
      mask Display:
      | choice1 = get_param(gcb,'JJoint');
      | color('black');
      | switch choice1
      |     case '1'
      |         disp('获取关节1电机\n外转子角度(rad)');
      |     case '2'
      |         disp('获取关节2电机\n外转子角度(rad)');
      |     case '3'
      |         disp('获取关节3电机\n外转子角度(rad)');
      |     case '4'
      |         disp('获取关节4电机\n外转子角度(rad)');
      |     case '5'
      |         disp('获取关节5电机\n外转子角度(rad)');
      |     case '6'
      |         disp('获取关节6电机\n外转子角度(rad)');
      | end
      | color('black');
      | port_label('output', 1, 'Angle');
      | port_label('output', 2, 'InitAngle');
      | clear choice1;
  GetAngle4 : Subsystem  TreatAsAtomicUnit=on  mask(获取电机外转子角度(rad)){JJoint=4, InitAngle=0}
      mask prompts: JJoint "选择关节电机"; InitAngle "给定初始角度(deg)"
      mask help:
      | 给定初始角度：假设在数学建模时，设定连杆在水平位置为0°，而机械臂每个关节在出厂时都设定在竖直位置为0°，那么这里就需要给定一个偏置值90°/-90°，默认设为0。
      | 注：关节3因为结构原因实际获取到的角度的正负和标签贴的方向相反。
      | Angle(rad)=电机外转子的实际角度值-给定的初始角度值
      | InitAngle(rad)=给定的初始角度值
      mask TypeOptions JJoint: 1 | 2 | 3 | 4 | 5 | 6
      mask Display:
      | choice1 = get_param(gcb,'JJoint');
      | color('black');
      | switch choice1
      |     case '1'
      |         disp('获取关节1电机\n外转子角度(rad)');
      |     case '2'
      |         disp('获取关节2电机\n外转子角度(rad)');
      |     case '3'
      |         disp('获取关节3电机\n外转子角度(rad)');
      |     case '4'
      |         disp('获取关节4电机\n外转子角度(rad)');
      |     case '5'
      |         disp('获取关节5电机\n外转子角度(rad)');
      |     case '6'
      |         disp('获取关节6电机\n外转子角度(rad)');
      | end
      | color('black');
      | port_label('output', 1, 'Angle');
      | port_label('output', 2, 'InitAngle');
      | clear choice1;
  GetAngle5 : Subsystem  TreatAsAtomicUnit=on  mask(获取电机外转子角度(rad)){JJoint=5, InitAngle=0}
      mask prompts: JJoint "选择关节电机"; InitAngle "给定初始角度(deg)"
      mask help:
      | 给定初始角度：假设在数学建模时，设定连杆在水平位置为0°，而机械臂每个关节在出厂时都设定在竖直位置为0°，那么这里就需要给定一个偏置值90°/-90°，默认设为0。
      | 注：关节3因为结构原因实际获取到的角度的正负和标签贴的方向相反。
      | Angle(rad)=电机外转子的实际角度值-给定的初始角度值
      | InitAngle(rad)=给定的初始角度值
      mask TypeOptions JJoint: 1 | 2 | 3 | 4 | 5 | 6
      mask Display:
      | choice1 = get_param(gcb,'JJoint');
      | color('black');
      | switch choice1
      |     case '1'
      |         disp('获取关节1电机\n外转子角度(rad)');
      |     case '2'
      |         disp('获取关节2电机\n外转子角度(rad)');
      |     case '3'
      |         disp('获取关节3电机\n外转子角度(rad)');
      |     case '4'
      |         disp('获取关节4电机\n外转子角度(rad)');
      |     case '5'
      |         disp('获取关节5电机\n外转子角度(rad)');
      |     case '6'
      |         disp('获取关节6电机\n外转子角度(rad)');
      | end
      | color('black');
      | port_label('output', 1, 'Angle');
      | port_label('output', 2, 'InitAngle');
      | clear choice1;
  GetAngle6 : Subsystem  TreatAsAtomicUnit=on  mask(获取电机外转子角度(rad)){JJoint=6, InitAngle=0}
      mask prompts: JJoint "选择关节电机"; InitAngle "给定初始角度(deg)"
      mask help:
      | 给定初始角度：假设在数学建模时，设定连杆在水平位置为0°，而机械臂每个关节在出厂时都设定在竖直位置为0°，那么这里就需要给定一个偏置值90°/-90°，默认设为0。
      | 注：关节3因为结构原因实际获取到的角度的正负和标签贴的方向相反。
      | Angle(rad)=电机外转子的实际角度值-给定的初始角度值
      | InitAngle(rad)=给定的初始角度值
      mask TypeOptions JJoint: 1 | 2 | 3 | 4 | 5 | 6
      mask Display:
      | choice1 = get_param(gcb,'JJoint');
      | color('black');
      | switch choice1
      |     case '1'
      |         disp('获取关节1电机\n外转子角度(rad)');
      |     case '2'
      |         disp('获取关节2电机\n外转子角度(rad)');
      |     case '3'
      |         disp('获取关节3电机\n外转子角度(rad)');
      |     case '4'
      |         disp('获取关节4电机\n外转子角度(rad)');
      |     case '5'
      |         disp('获取关节5电机\n外转子角度(rad)');
      |     case '6'
      |         disp('获取关节6电机\n外转子角度(rad)');
      | end
      | color('black');
      | port_label('output', 1, 'Angle');
      | port_label('output', 2, 'InitAngle');
      | clear choice1;
  GetAngleSpeed : Subsystem  Priority=2  TreatAsAtomicUnit=on  mask{JJoint=1}
      mask prompts: JJoint "选择关节电机"
      mask help: 读取电机角速度(rad/s)
      mask TypeOptions JJoint: 1 | 2 | 3 | 4 | 5 | 6
      mask Display:
      | choice1 = get_param(gcb,'JJoint');
      | color('black');
      | switch choice1
      |     case '1'
      |         disp('获取关节1电机\n外转子角速度(rad/s)');
      |     case '2'
      |         disp('获取关节2电机\n外转子角速度(rad/s)');
      |     case '3'
      |         disp('获取关节3电机\n外转子角速度(rad/s)');
      |     case '4'
      |         disp('获取关节4电机\n外转子角速度(rad/s)');
      |     case '5'
      |         disp('获取关节5电机\n外转子角速度(rad/s)');
      |     case '6'
      |         disp('获取关节6电机\n外转子角速度(rad/s)');
      | end
      | color('black');
      | port_label('output', 1, 'Velocity');
      | clear choice1;
  GetAngleSpeed1 : Subsystem  Priority=2  TreatAsAtomicUnit=on  mask{JJoint=2}
      mask prompts: JJoint "选择关节电机"
      mask help: 读取电机角速度(rad/s)
      mask TypeOptions JJoint: 1 | 2 | 3 | 4 | 5 | 6
      mask Display:
      | choice1 = get_param(gcb,'JJoint');
      | color('black');
      | switch choice1
      |     case '1'
      |         disp('获取关节1电机\n外转子角速度(rad/s)');
      |     case '2'
      |         disp('获取关节2电机\n外转子角速度(rad/s)');
      |     case '3'
      |         disp('获取关节3电机\n外转子角速度(rad/s)');
      |     case '4'
      |         disp('获取关节4电机\n外转子角速度(rad/s)');
      |     case '5'
      |         disp('获取关节5电机\n外转子角速度(rad/s)');
      |     case '6'
      |         disp('获取关节6电机\n外转子角速度(rad/s)');
      | end
      | color('black');
      | port_label('output', 1, 'Velocity');
      | clear choice1;
  GetAngleSpeed2 : Subsystem  Priority=2  TreatAsAtomicUnit=on  mask{JJoint=3}
      mask prompts: JJoint "选择关节电机"
      mask help: 读取电机角速度(rad/s)
      mask TypeOptions JJoint: 1 | 2 | 3 | 4 | 5 | 6
      mask Display:
      | choice1 = get_param(gcb,'JJoint');
      | color('black');
      | switch choice1
      |     case '1'
      |         disp('获取关节1电机\n外转子角速度(rad/s)');
      |     case '2'
      |         disp('获取关节2电机\n外转子角速度(rad/s)');
      |     case '3'
      |         disp('获取关节3电机\n外转子角速度(rad/s)');
      |     case '4'
      |         disp('获取关节4电机\n外转子角速度(rad/s)');
      |     case '5'
      |         disp('获取关节5电机\n外转子角速度(rad/s)');
      |     case '6'
      |         disp('获取关节6电机\n外转子角速度(rad/s)');
      | end
      | color('black');
      | port_label('output', 1, 'Velocity');
      | clear choice1;
  GetAngleSpeed3 : Subsystem  Priority=2  TreatAsAtomicUnit=on  mask{JJoint=4}
      mask prompts: JJoint "选择关节电机"
      mask help: 读取电机角速度(rad/s)
      mask TypeOptions JJoint: 1 | 2 | 3 | 4 | 5 | 6
      mask Display:
      | choice1 = get_param(gcb,'JJoint');
      | color('black');
      | switch choice1
      |     case '1'
      |         disp('获取关节1电机\n外转子角速度(rad/s)');
      |     case '2'
      |         disp('获取关节2电机\n外转子角速度(rad/s)');
      |     case '3'
      |         disp('获取关节3电机\n外转子角速度(rad/s)');
      |     case '4'
      |         disp('获取关节4电机\n外转子角速度(rad/s)');
      |     case '5'
      |         disp('获取关节5电机\n外转子角速度(rad/s)');
      |     case '6'
      |         disp('获取关节6电机\n外转子角速度(rad/s)');
      | end
      | color('black');
      | port_label('output', 1, 'Velocity');
      | clear choice1;
  GetAngleSpeed4 : Subsystem  Priority=2  TreatAsAtomicUnit=on  mask{JJoint=5}
      mask prompts: JJoint "选择关节电机"
      mask help: 读取电机角速度(rad/s)
      mask TypeOptions JJoint: 1 | 2 | 3 | 4 | 5 | 6
      mask Display:
      | choice1 = get_param(gcb,'JJoint');
      | color('black');
      | switch choice1
      |     case '1'
      |         disp('获取关节1电机\n外转子角速度(rad/s)');
      |     case '2'
      |         disp('获取关节2电机\n外转子角速度(rad/s)');
      |     case '3'
      |         disp('获取关节3电机\n外转子角速度(rad/s)');
      |     case '4'
      |         disp('获取关节4电机\n外转子角速度(rad/s)');
      |     case '5'
      |         disp('获取关节5电机\n外转子角速度(rad/s)');
      |     case '6'
      |         disp('获取关节6电机\n外转子角速度(rad/s)');
      | end
      | color('black');
      | port_label('output', 1, 'Velocity');
      | clear choice1;
  GetAngleSpeed5 : Subsystem  Priority=2  TreatAsAtomicUnit=on  mask{JJoint=6}
      mask prompts: JJoint "选择关节电机"
      mask help: 读取电机角速度(rad/s)
      mask TypeOptions JJoint: 1 | 2 | 3 | 4 | 5 | 6
      mask Display:
      | choice1 = get_param(gcb,'JJoint');
      | color('black');
      | switch choice1
      |     case '1'
      |         disp('获取关节1电机\n外转子角速度(rad/s)');
      |     case '2'
      |         disp('获取关节2电机\n外转子角速度(rad/s)');
      |     case '3'
      |         disp('获取关节3电机\n外转子角速度(rad/s)');
      |     case '4'
      |         disp('获取关节4电机\n外转子角速度(rad/s)');
      |     case '5'
      |         disp('获取关节5电机\n外转子角速度(rad/s)');
      |     case '6'
      |         disp('获取关节6电机\n外转子角速度(rad/s)');
      | end
      | color('black');
      | port_label('output', 1, 'Velocity');
      | clear choice1;
  Mux : Mux  Inputs=6
  Mux1 : Mux  Inputs=6
  Mux2 : Mux  Inputs=6
  q(rad) : Outport
  InitAngle(rad) : Outport  Port=2
  q_dot(rad/s) : Outport  Port=3
  wires:
  GetAngle4/1(Angle) -> Mux/4
  GetAngle3/1(Angle) -> Mux/3
  GetAngle5/1(Angle) -> Mux/5
  GetAngle1/1(Angle) -> Mux/1
  GetAngle2/1(Angle) -> Mux/2
  GetAngle6/1(Angle) -> Mux/6
  Mux/1 -> q(rad)/1
  GetAngleSpeed/1(Velcity) -> Mux1/1
  GetAngleSpeed1/1(Velcity) -> Mux1/2
  GetAngleSpeed2/1(Velcity) -> Mux1/3
  GetAngleSpeed3/1(Velcity) -> Mux1/4
  GetAngleSpeed4/1(Velcity) -> Mux1/5
  GetAngleSpeed5/1(Velcity) -> Mux1/6
  Mux1/1 -> q_dot(rad/s)/1
  GetAngle1/2(InitAngle) -> Mux2/1
  GetAngle2/2(InitAngle) -> Mux2/2
  GetAngle3/2(InitAngle) -> Mux2/3
  GetAngle4/2(InitAngle) -> Mux2/4
  GetAngle5/2(InitAngle) -> Mux2/5
  GetAngle6/2(InitAngle) -> Mux2/6
  Mux2/1 -> InitAngle(rad)/1

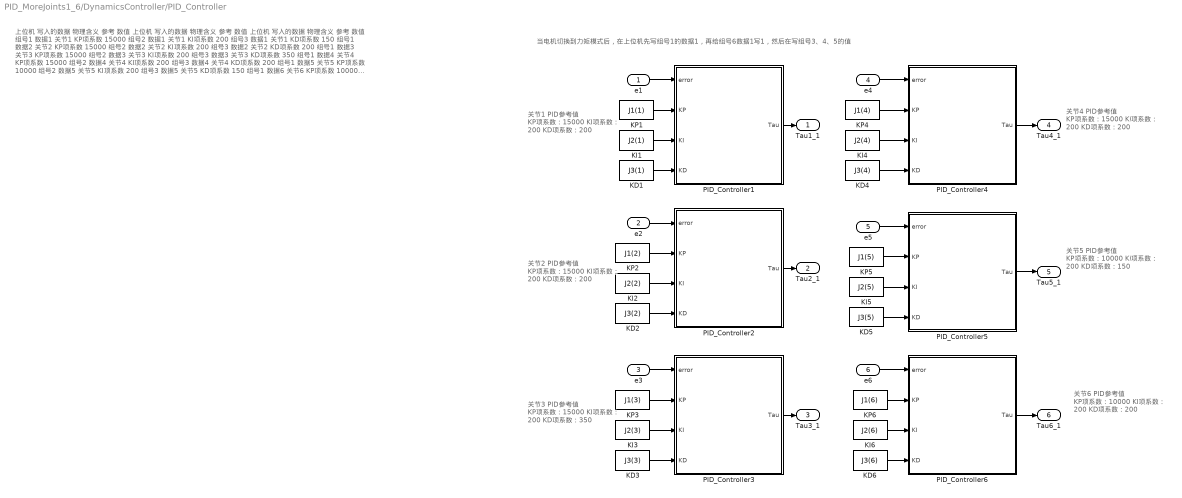
== system PID_MoreJoints1_6/DynamicsController/PID_Controller ==
  note: 上位机
      | 写入的数据
      | 物理含义
      | 参考
      | 数值
      | 上位机
      | 写入的数据
      | 物理含义
      | 参考
      | 数值
      | 上位机
      | 写入的数据
      | 物理含义
      | 参考
      | 数值
      |
      | 组号1
      | 数据1
      | 关节1
      | KP项系数
      | 15000
      | 组号2
      | 数据1
      | 关节1
      | KI项系数
      | 200
      | 组号3
      | 数据1
      | 关节1
      | KD项系数
      | 150
      |
      | 组号1
      | 数据2
      | 关节2
      | KP项系数
      | 15000
      | 组号2
      | 数据2
      | 关节2
      | KI项系数
      | 200
      | 组号3
      | 数据2
      | 关节2
      | KD项系数
      | 200
      |
      | 组号1
      | 数据3
      | 关节3
      | KP项系数
      | 15000
      | 组号2
      | 数据3
      | 关节3
      | KI项系数
      | 200
      | 组号3
      | 数据3
      | 关节3
      | KD项系数
      | 350
      |
      | 组号1
      | 数据4
      | 关节4
      | KP项系数
      | 15000
      | 组号2
      | 数据4
      | 关节4
      | KI项系数
      | 200
      | 组号3
      | 数据4
      | 关节4
      | KD项系数
      | 200
      |
      | 组号1
      | 数据5
      | 关节5
      | KP项系数
      | 10000
      | 组号2
      | 数据5
      | 关节5
      | KI项系数
      | 200
      | 组号3
      | 数据5
      | 关节5
      | KD项系数
      | 150
      |
      | 组号1
      | 数据6
      | 关节6
      | KP项系数
      | 10000
      | 组号2
      | 数据6
      | 关节6
      | KI项系数
      | 200
      | 组号3
      | 数据6
      | 关节6
      | KD项系数
      | 200
      |
      | 上位机
      | 写入的数据
      | 物理含义
      | 参考
      | 数值
      | 上位机
      | 写入的数据
      | 物理含义
      | 参考
      | 数值
      | 上位机
      | 写入的数据
      | 物理含义
      | 参考
      | 数值
      |
      | 组号4
      | 数据1
      | 关节2库伦摩擦力系数
      | 20
      | 组号5
      | 数据1
      | 关节1库伦摩擦力系数
      | 30
      | 组号6
      | 数据1
      | 所有关节正弦信号使能开关
      | 1
      |
      | 组号4
      | 数据2
      | 关节2黏性摩擦力系数
      | 80
      | 组号5
      | 数据2
      | 关节1黏性摩擦力系数
      | 60
      | 组号6
      | 数据2
      |
      | 组号4
      | 数据3
      | 关节3库伦摩擦力系数
      | 20
      | 组号5
      | 数据3
      | 关节5库伦摩擦力系数
      | 15
      | 组号6
      | 数据3
      |
      | 组号4
      | 数据4
      | 关节3黏性摩擦力系数
      | 75
      | 组号5
      | 数据4
      | 关节5黏性摩擦力系数
      | 30
      | 组号6
      | 数据4
      |
      | 组号4
      | 数据5
      | 关节4库伦摩擦力系数
      | 10
      | 组号5
      | 数据5
      | 关节6库伦摩擦力系数
      | 10
      | 组号6
      | 数据5
      |
      | 组号4
      | 数据6
      | 关节4黏性摩擦力系数
      | 30
      | 组号5
      | 数据6
      | 关节6黏性摩擦力系数
      | 50
      | 组号6
      | 数据6
  note: 当电机切换到力矩模式后，在上位机先写组号1的数据1，再给组号6数据1写1，然后在写组号3、4、5的值
  note: 关节3 PID参考值
      | KP项系数：15000
      | KI项系数： 200
      | KD项系数：350
  note: 关节5 PID参考值
      | KP项系数：10000
      | KI项系数： 200
      | KD项系数：150
  note: 关节2 PID参考值
      | KP项系数：15000
      | KI项系数： 200
      | KD项系数：200
  note: 关节4 PID参考值
      | KP项系数：15000
      | KI项系数： 200
      | KD项系数：200
  note: 关节6 PID参考值
      | KP项系数：10000
      | KI项系数： 200
      | KD项系数：200
  note: 关节1 PID参考值
      | KP项系数：15000
      | KI项系数： 200
      | KD项系数：200
  e1 : Inport
  e2 : Inport  Port=2
  e3 : Inport  Port=3
  e4 : Inport  Port=4
  e5 : Inport  Port=5
  e6 : Inport  Port=6
  KD1 : DataStoreRead  DataStoreName=J3  DataStoreElements=J3(1)
  KD2 : DataStoreRead  DataStoreName=J3  DataStoreElements=J3(2)
  KD3 : DataStoreRead  DataStoreName=J3  DataStoreElements=J3(3)
  KD4 : DataStoreRead  DataStoreName=J3  DataStoreElements=J3(4)
  KD5 : DataStoreRead  DataStoreName=J3  DataStoreElements=J3(5)
  KD6 : DataStoreRead  DataStoreName=J3  DataStoreElements=J3(6)
  KI1 : DataStoreRead  DataStoreName=J2  DataStoreElements=J2(1)
  KI2 : DataStoreRead  DataStoreName=J2  DataStoreElements=J2(2)
  KI3 : DataStoreRead  DataStoreName=J2  DataStoreElements=J2(3)
  KI4 : DataStoreRead  DataStoreName=J2  DataStoreElements=J2(4)
  KI5 : DataStoreRead  DataStoreName=J2  DataStoreElements=J2(5)
  KI6 : DataStoreRead  DataStoreName=J2  DataStoreElements=J2(6)
  KP1 : DataStoreRead  DataStoreName=J1  DataStoreElements=J1(1)
  KP2 : DataStoreRead  DataStoreName=J1  DataStoreElements=J1(2)
  KP3 : DataStoreRead  DataStoreName=J1  DataStoreElements=J1(3)
  KP4 : DataStoreRead  DataStoreName=J1  DataStoreElements=J1(4)
  KP5 : DataStoreRead  DataStoreName=J1  DataStoreElements=J1(5)
  KP6 : DataStoreRead  DataStoreName=J1  DataStoreElements=J1(6)
  PID_Controller1 : Subsystem  TreatAsAtomicUnit=on
  PID_Controller2 : Subsystem  TreatAsAtomicUnit=on
  PID_Controller3 : Subsystem  TreatAsAtomicUnit=on
  PID_Controller4 : Subsystem  TreatAsAtomicUnit=on
  PID_Controller5 : Subsystem  TreatAsAtomicUnit=on
  PID_Controller6 : Subsystem  TreatAsAtomicUnit=on
  Tau1_1 : Outport
  Tau2_1 : Outport  Port=2
  Tau3_1 : Outport  Port=3
  Tau4_1 : Outport  Port=4
  Tau5_1 : Outport  Port=5
  Tau6_1 : Outport  Port=6
  wires:
  KD5/1 -> PID_Controller5/4(KD)
  KP5/1 -> PID_Controller5/2(KP)
  KI5/1 -> PID_Controller5/3(KI)
  e5/1 -> PID_Controller5/1(error)
  PID_Controller5/1(Tau) -> Tau5_1/1
  e1/1 -> PID_Controller1/1(error)
  PID_Controller1/1(Tau) -> Tau1_1/1
  PID_Controller2/1(Tau) -> Tau2_1/1
  PID_Controller3/1(Tau) -> Tau3_1/1
  PID_Controller4/1(Tau) -> Tau4_1/1
  PID_Controller6/1(Tau) -> Tau6_1/1
  e2/1 -> PID_Controller2/1(error)
  e3/1 -> PID_Controller3/1(error)
  e4/1 -> PID_Controller4/1(error)
  e6/1 -> PID_Controller6/1(error)
  KP1/1 -> PID_Controller1/2(KP)
  KP2/1 -> PID_Controller2/2(KP)
  KP3/1 -> PID_Controller3/2(KP)
  KP6/1 -> PID_Controller6/2(KP)
  KI6/1 -> PID_Controller6/3(KI)
  KD6/1 -> PID_Controller6/4(KD)
  KP4/1 -> PID_Controller4/2(KP)
  KD4/1 -> PID_Controller4/4(KD)
  KD3/1 -> PID_Controller3/4(KD)
  KD1/1 -> PID_Controller1/4(KD)
  KD2/1 -> PID_Controller2/4(KD)
  KI1/1 -> PID_Controller1/3(KI)
  KI2/1 -> PID_Controller2/3(KI)
  KI4/1 -> PID_Controller4/3(KI)
  KI3/1 -> PID_Controller3/3(KI)

== system PID_MoreJoints1_6/DynamicsController/关节一正弦信号发生器 ==
  note: 0~60
  En : Inport
  q : Inport  Port=2
  Constant3 : Constant  Value=20
  Gain14 : Gain  Gain=pi/180
  Subsystem : Subsystem  mask(单关节正弦信号生产器){Freq=1/4, SimpleTime=0.001}
      mask prompts: Freq "正弦信号的频率(HZ)"; SimpleTime "正弦信号的采样时间(s)"
      mask help:
      | 采样频率不能过快，否则机械臂摆动频率也会变快，至少为1/4.
      | 采样时间只能是定时器步长的整数倍，否则会报错。
      mask Display:
      | color('red');
      | disp('单关节正弦信号发生器');
      | color('black');
      | port_label('input', 1, '外转子实际角度(rad)');
      | port_label('input', 2, '外转子正弦信号的幅值');
      | port_label('Enable','Enable')
      | port_label('output', 1, '外转子理想正弦信号');
      | port_label('output', 2, '外转子跟踪误差(rad)');
  qd : Outport
  e : Outport  Port=2
  wires:
  Subsystem/1(外转子理想 正弦信号) -> qd/1
  Constant3/1 -> Gain14/1
  Subsystem/2(电机外转子 跟踪误差) -> e/1
  Gain14/1 -> Subsystem/2(电机外转子 正弦信号的幅值)
  En/1 -> Subsystem/Enable
  q/1 -> Subsystem/1(电机外转子 实际角度(rad))

== system PID_MoreJoints1_6/DynamicsController/关节三正弦信号发生器 ==
  note: 0~60
  En : Inport
  q : Inport  Port=2
  Constant3 : Constant  Value=20
  Gain14 : Gain  Gain=pi/180
  Subsystem : Subsystem  mask(单关节正弦信号生产器){Freq=1/4, SimpleTime=0.001}
      mask prompts: Freq "正弦信号的频率(HZ)"; SimpleTime "正弦信号的采样时间(s)"
      mask help:
      | 采样频率不能过快，否则机械臂摆动频率也会变快，至少为1/4.
      | 采样时间只能是定时器步长的整数倍，否则会报错。
      mask Display:
      | color('red');
      | disp('单关节正弦信号发生器');
      | color('black');
      | port_label('input', 1, '外转子实际角度(rad)');
      | port_label('input', 2, '外转子正弦信号的幅值');
      | port_label('Enable','Enable')
      | port_label('output', 1, '外转子理想正弦信号');
      | port_label('output', 2, '外转子跟踪误差(rad)');
  qd : Outport
  e : Outport  Port=2
  wires:
  Subsystem/1(外转子理想 正弦信号) -> qd/1
  Constant3/1 -> Gain14/1
  Subsystem/2(电机外转子 跟踪误差) -> e/1
  Gain14/1 -> Subsystem/2(电机外转子 正弦信号的幅值)
  En/1 -> Subsystem/Enable
  q/1 -> Subsystem/1(电机外转子 实际角度(rad))

== system PID_MoreJoints1_6/DynamicsController/关节二正弦信号发生器 ==
  note: 0~60
  En : Inport
  q : Inport  Port=2
  Constant3 : Constant  Value=20
  Gain14 : Gain  Gain=pi/180
  Subsystem : Subsystem  mask(单关节正弦信号生产器){Freq=1/4, SimpleTime=0.001}
      mask prompts: Freq "正弦信号的频率(HZ)"; SimpleTime "正弦信号的采样时间(s)"
      mask help:
      | 采样频率不能过快，否则机械臂摆动频率也会变快，至少为1/4.
      | 采样时间只能是定时器步长的整数倍，否则会报错。
      mask Display:
      | color('red');
      | disp('单关节正弦信号发生器');
      | color('black');
      | port_label('input', 1, '外转子实际角度(rad)');
      | port_label('input', 2, '外转子正弦信号的幅值');
      | port_label('Enable','Enable')
      | port_label('output', 1, '外转子理想正弦信号');
      | port_label('output', 2, '外转子跟踪误差(rad)');
  qd : Outport
  e : Outport  Port=2
  wires:
  q/1 -> Subsystem/1(电机外转子 实际角度(rad))
  En/1 -> Subsystem/Enable
  Gain14/1 -> Subsystem/2(电机外转子 正弦信号的幅值)
  Subsystem/2(电机外转子 跟踪误差) -> e/1
  Constant3/1 -> Gain14/1
  Subsystem/1(外转子理想 正弦信号) -> qd/1

== system PID_MoreJoints1_6/DynamicsController/关节五正弦信号发生器 ==
  note: 0~60
  En : Inport
  q : Inport  Port=2
  Constant3 : Constant  Value=20
  Gain14 : Gain  Gain=pi/180
  Subsystem : Subsystem  mask(单关节正弦信号生产器){Freq=1/4, SimpleTime=0.001}
      mask prompts: Freq "正弦信号的频率(HZ)"; SimpleTime "正弦信号的采样时间(s)"
      mask help:
      | 采样频率不能过快，否则机械臂摆动频率也会变快，至少为1/4.
      | 采样时间只能是定时器步长的整数倍，否则会报错。
      mask Display:
      | color('red');
      | disp('单关节正弦信号发生器');
      | color('black');
      | port_label('input', 1, '外转子实际角度(rad)');
      | port_label('input', 2, '外转子正弦信号的幅值');
      | port_label('Enable','Enable')
      | port_label('output', 1, '外转子理想正弦信号');
      | port_label('output', 2, '外转子跟踪误差(rad)');
  qd : Outport
  e : Outport  Port=2
  wires:
  Subsystem/1(外转子理想 正弦信号) -> qd/1
  Constant3/1 -> Gain14/1
  Subsystem/2(电机外转子 跟踪误差) -> e/1
  Gain14/1 -> Subsystem/2(电机外转子 正弦信号的幅值)
  En/1 -> Subsystem/Enable
  q/1 -> Subsystem/1(电机外转子 实际角度(rad))
